simulink model "system_7d"  (Simulink 8.6)
settings: Solver=VariableStepAuto  StartTime=0.0  StopTime=10.0  RelTol=1e-3
libraries: simulink x1
settings Model: Creator=xinchen  LastModifiedBy=xinchen
settings DataIOCC: SaveFormat=Dataset  SignalLoggingSaveFormat=Dataset
settings OptimizationCC: ExpressionDepthLimit=128
settings DebuggingCC: UnderspecifiedInitializationDetection=Simplified  MergeDetectMultiDrivingBlocksExec=error  SolverPrmCheckMsg=none  FcnCallInpInsideContextMsg=EnableAllAsError  StateNameClashWarn=none
settings HardwareCC: ProdBitPerPointer=64  ProdLargestAtomicFloat=Float  ProdIntDivRoundTo=Zero  ProdEndianess=LittleEndian  ProdWordSize=64  ProdHWDeviceType=Intel->x86-64 (Windows64)
settings GRTTargetCC: GeneratePreprocessorConditionals=Use local settings  CombineOutputUpdateFcns=on  GRTInterface=off
settings ConfigComp: CovModelRefEnable=off

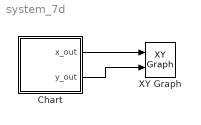
== system system_7d ==
  Chart : Stateflow chart  TreatAsAtomicUnit=on
  XY Graph : simulink/Sinks/XY Graph  xmin=0  xmax=1.2  ymin=0.15  ymax=0.5  st=0.01
  wires:
  Chart/1(x_out) -> XY Graph/1
  Chart/2(y_out) -> XY Graph/2

== stateflow chart Chart ==
  settings: updateMethod=CONTINUOUS
  state VO
    du:
    x1_dot = 1.4*x3-0.9*x1;
    x2_dot = 2.5*x5-1.5*x2;
    x3_dot = 0.6*x7-0.8*x3*x2;
    x4_dot = 2.0-1.3*x4*x3;
    x5_dot = 0.7*x1-1.0*x4*x5;
    x6_dot = 0.3*x1-3.1*x6;
    x7_dot = 1.8*x6-1.5*x7*x2;
    x_out = x5;
    y_out = x7;
  note: @annotation-mode=VO;
      | k=2000;
      | gamma=0;
  (default) -> VO : {x1=1.2; x2=1.05;x3=1.5;x4=2.4;x5=1.0;x6=0.1;x7=0.45;}
  data: x_out output double; y_out output double; x1 local double; x2 local double; x3 local double; x4 local double; x5 local double; x6 local double; x7 local double
  data x1 settings: updateMethod=SF_CONTINUOUS_TIME_DATA
  data x2 settings: updateMethod=SF_CONTINUOUS_TIME_DATA
  data x3 settings: updateMethod=SF_CONTINUOUS_TIME_DATA
  data x4 settings: updateMethod=SF_CONTINUOUS_TIME_DATA
  data x5 settings: updateMethod=SF_CONTINUOUS_TIME_DATA
  data x6 settings: updateMethod=SF_CONTINUOUS_TIME_DATA
  data x7 settings: updateMethod=SF_CONTINUOUS_TIME_DATA
